simulink model "part_m"  (R2022b)
settings: Solver=ode4  StartTime=0.0  StopTime=inf  FixedStep=0.002  RelTol=1e-3
InitFcn:
  | init; % init script
values from neighbouring files (symbols this model uses):
  attitude_m0 = [theta_m0; psi_m0]    [init.m]
  attitude_t0 = [theta_t0; psi_t0]    [init.m]
  d_state_m = T_VG_m'*[V_m0;0;0;]    [init.m]
  d_state_t = T_VG_t'*[V_t0;0;0;]    [init.m]
  k_epsilon_lead_angle = k(1)    [init.m]
  k_sigma_lead_angle = k(2)    [init.m]
  state_m0 = [x_m0; y_m0; z_m0]    [init.m]
  state_t0 = [x_t0; y_t0; z_t0]    [init.m]
libraries: simulink x3
(part 1 of 2)
settings Model: Creator=Ali  LastModifiedBy=Ali

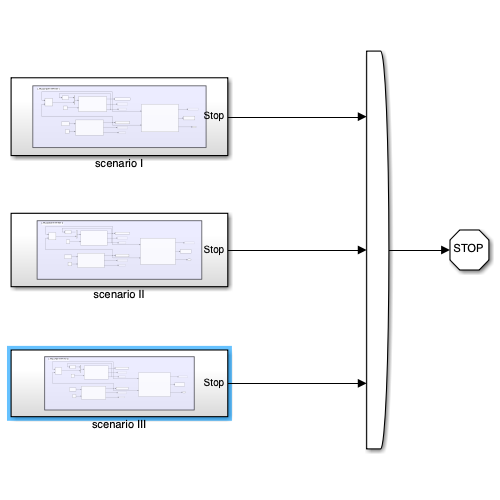
[thumbnail: Simulink's stored preview of the top-level diagram]
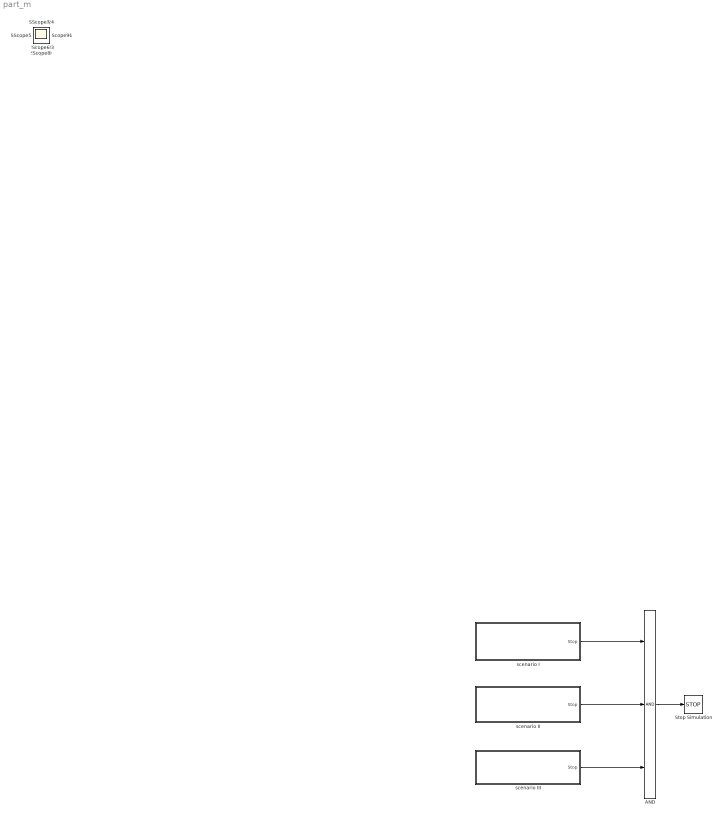
== system part_m ==
  AND : Logic  Inputs=3  IconShape=distinctive  AllPortsSameDT=off  OutDataTypeStr=boolean
  Stop Simulation : Stop
  scenario I : Subsystem
  scenario II : Subsystem
  scenario III : Subsystem
  Scope{,1..18,20..24} (24 alike) : Scope
  wires:
  scenario I/1(Stop) -> AND/1
  scenario II/1(Stop) -> AND/2
  scenario III/1(Stop) -> AND/3
  AND/1 -> Stop Simulation/1

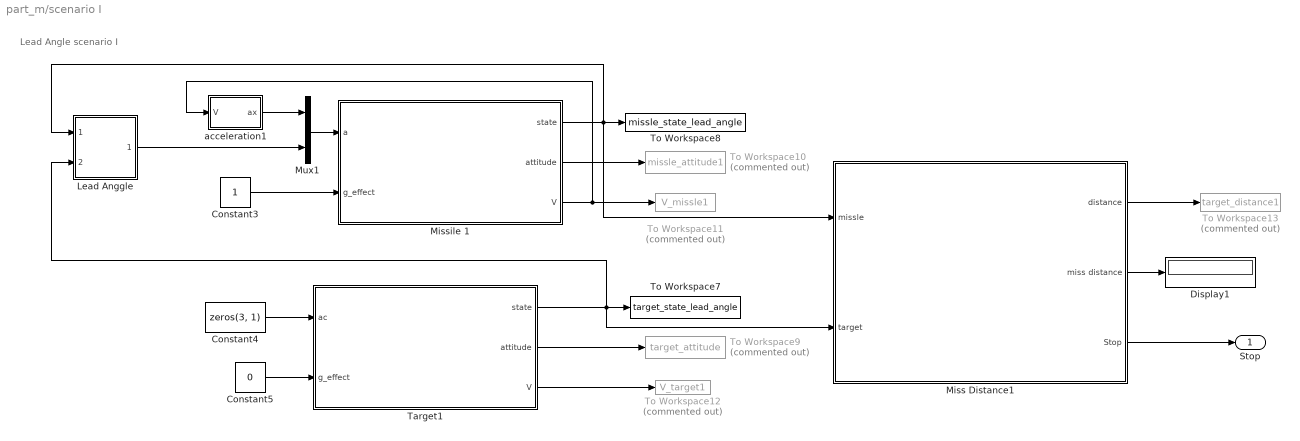
== system part_m/scenario I ==
  note: Lead Angle scenario I
  Constant3 : Constant
  Constant4 : Constant  Value=zeros(3, 1)
  Constant5 : Constant  Value=0
  Display1 : Display
  Lead Anggle : Subsystem
  Miss Distance1 : Subsystem
  Missile 1 : Subsystem
  Mux1 : Mux  Inputs=2
  Target1 : Subsystem
  To Workspace10 : ToWorkspace  Commented=on  VariableName=missle_attitude1  SaveFormat=Timeseries  SampleTime=-1
      settings: Save2DSignal=2-D array (concatenate along first dimension)
  To Workspace11 : ToWorkspace  Commented=on  VariableName=V_missle1  SaveFormat=Timeseries  SampleTime=-1
      settings: Save2DSignal=2-D array (concatenate along first dimension)
  To Workspace12 : ToWorkspace  Commented=on  VariableName=V_target1  SaveFormat=Timeseries  SampleTime=-1
      settings: Save2DSignal=2-D array (concatenate along first dimension)
  To Workspace13 : ToWorkspace  Commented=on  VariableName=target_distance1  SaveFormat=Timeseries  SampleTime=-1
      settings: Save2DSignal=2-D array (concatenate along first dimension)
  To Workspace7 : ToWorkspace  VariableName=target_state_lead_angle  SaveFormat=Timeseries  SampleTime=-1
      settings: Save2DSignal=2-D array (concatenate along first dimension)
  To Workspace8 : ToWorkspace  VariableName=missle_state_lead_angle  SaveFormat=Timeseries  SampleTime=-1
      settings: Save2DSignal=2-D array (concatenate along first dimension)
  To Workspace9 : ToWorkspace  Commented=on  VariableName=target_attitude  SaveFormat=Timeseries  SampleTime=-1
      settings: Save2DSignal=2-D array (concatenate along first dimension)
  acceleration1 : Subsystem
  Stop : Outport
  wires:
  acceleration1/1(ax) -> Mux1/1
  Miss Distance1/2(miss distance) -> Display1/1
  Constant4/1 -> Target1/1(ac)
  Constant3/1 -> Missile 1/2(g_effect)
  Lead Anggle/1("ay, az") -> Mux1/2
  Mux1/1 -> Missile 1/1(a)
  Constant5/1 -> Target1/2(g_effect)
  Missile 1/2(attitude) -> To Workspace10/1
  Target1/1(state) -> Lead Anggle/2(target_state), Miss Distance1/2(target), To Workspace7/1
  Target1/2(attitude) -> To Workspace9/1
  Missile 1/1(state) -> Lead Anggle/1(missle_state), Miss Distance1/1(missle), To Workspace8/1
  Miss Distance1/3(Stop) -> Stop/1
  Target1/3(V) -> To Workspace12/1
  Miss Distance1/1(distance) -> To Workspace13/1
  Missile 1/3(V) -> acceleration1/1(V), To Workspace11/1

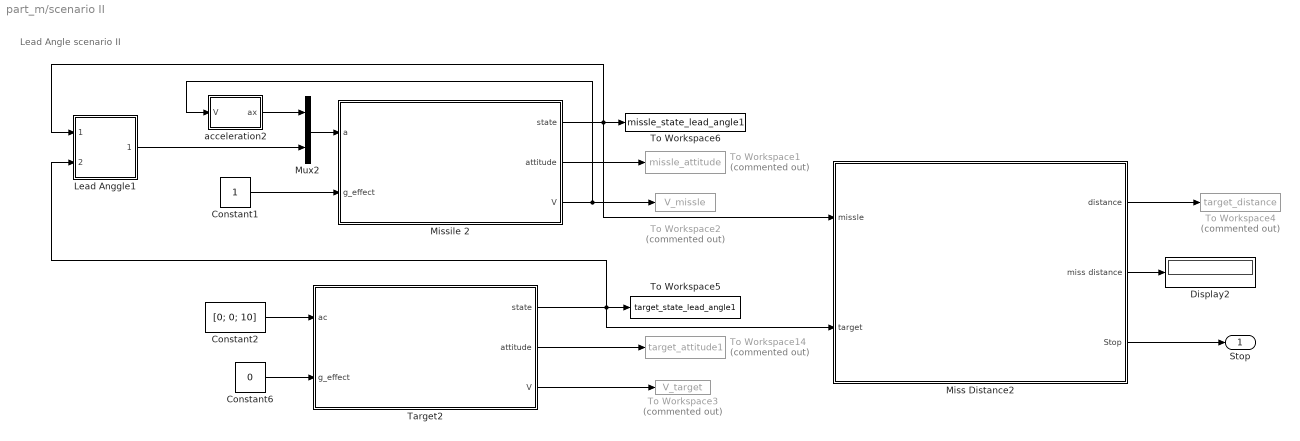
== system part_m/scenario II ==
  note: Lead Angle scenario II
  Constant1 : Constant
  Constant2 : Constant  Value=[0; 0; 10]
  Constant6 : Constant  Value=0
  Display2 : Display
  Lead Anggle1 : Subsystem
  Miss Distance2 : Subsystem
  Missile 2 : Subsystem
  Mux2 : Mux  Inputs=2
  Target2 : Subsystem
  To Workspace1 : ToWorkspace  Commented=on  VariableName=missle_attitude  SaveFormat=Timeseries  SampleTime=-1
      settings: Save2DSignal=2-D array (concatenate along first dimension)
  To Workspace14 : ToWorkspace  Commented=on  VariableName=target_attitude1  SaveFormat=Timeseries  SampleTime=-1
      settings: Save2DSignal=2-D array (concatenate along first dimension)
  To Workspace2 : ToWorkspace  Commented=on  VariableName=V_missle  SaveFormat=Timeseries  SampleTime=-1
      settings: Save2DSignal=2-D array (concatenate along first dimension)
  To Workspace3 : ToWorkspace  Commented=on  VariableName=V_target  SaveFormat=Timeseries  SampleTime=-1
      settings: Save2DSignal=2-D array (concatenate along first dimension)
  To Workspace4 : ToWorkspace  Commented=on  VariableName=target_distance  SaveFormat=Timeseries  SampleTime=-1
      settings: Save2DSignal=2-D array (concatenate along first dimension)
  To Workspace5 : ToWorkspace  VariableName=target_state_lead_angle1  SaveFormat=Timeseries  SampleTime=-1
      settings: Save2DSignal=2-D array (concatenate along first dimension)
  To Workspace6 : ToWorkspace  VariableName=missle_state_lead_angle1  SaveFormat=Timeseries  SampleTime=-1
      settings: Save2DSignal=2-D array (concatenate along first dimension)
  acceleration2 : Subsystem
  Stop : Outport
  wires:
  Constant6/1 -> Target2/2(g_effect)
  Miss Distance2/3(Stop) -> Stop/1
  Mux2/1 -> Missile 2/1(a)
  Missile 2/2(attitude) -> To Workspace1/1
  Lead Anggle1/1("ay, az") -> Mux2/2
  Constant2/1 -> Target2/1(ac)
  acceleration2/1(ax) -> Mux2/1
  Missile 2/3(V) -> acceleration2/1(V), To Workspace2/1
  Target2/2(attitude) -> To Workspace14/1
  Target2/3(V) -> To Workspace3/1
  Miss Distance2/2(miss distance) -> Display2/1
  Constant1/1 -> Missile 2/2(g_effect)
  Missile 2/1(state) -> Lead Anggle1/1(missle_state), Miss Distance2/1(missle), To Workspace6/1
  Miss Distance2/1(distance) -> To Workspace4/1
  Target2/1(state) -> Lead Anggle1/2(target_state), Miss Distance2/2(target), To Workspace5/1

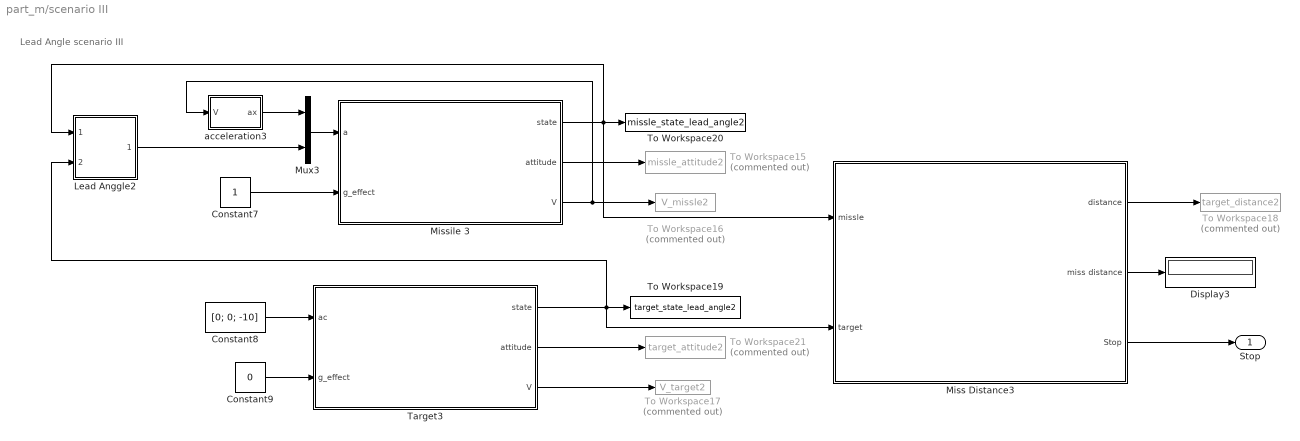
== system part_m/scenario III ==
  note: Lead Angle scenario III
  Constant7 : Constant
  Constant8 : Constant  Value=[0; 0; -10]
  Constant9 : Constant  Value=0
  Display3 : Display
  Lead Anggle2 : Subsystem
  Miss Distance3 : Subsystem
  Missile 3 : Subsystem
  Mux3 : Mux  Inputs=2
  Target3 : Subsystem
  To Workspace15 : ToWorkspace  Commented=on  VariableName=missle_attitude2  SaveFormat=Timeseries  SampleTime=-1
      settings: Save2DSignal=2-D array (concatenate along first dimension)
  To Workspace16 : ToWorkspace  Commented=on  VariableName=V_missle2  SaveFormat=Timeseries  SampleTime=-1
      settings: Save2DSignal=2-D array (concatenate along first dimension)
  To Workspace17 : ToWorkspace  Commented=on  VariableName=V_target2  SaveFormat=Timeseries  SampleTime=-1
      settings: Save2DSignal=2-D array (concatenate along first dimension)
  To Workspace18 : ToWorkspace  Commented=on  VariableName=target_distance2  SaveFormat=Timeseries  SampleTime=-1
      settings: Save2DSignal=2-D array (concatenate along first dimension)
  To Workspace19 : ToWorkspace  VariableName=target_state_lead_angle2  SaveFormat=Timeseries  SampleTime=-1
      settings: Save2DSignal=2-D array (concatenate along first dimension)
  To Workspace20 : ToWorkspace  VariableName=missle_state_lead_angle2  SaveFormat=Timeseries  SampleTime=-1
      settings: Save2DSignal=2-D array (concatenate along first dimension)
  To Workspace21 : ToWorkspace  Commented=on  VariableName=target_attitude2  SaveFormat=Timeseries  SampleTime=-1
      settings: Save2DSignal=2-D array (concatenate along first dimension)
  acceleration3 : Subsystem
  Stop : Outport
  wires:
  Miss Distance3/3(Stop) -> Stop/1
  Miss Distance3/1(distance) -> To Workspace18/1
  Target3/3(V) -> To Workspace17/1
  Target3/1(state) -> Lead Anggle2/2(target_state), Miss Distance3/2(target), To Workspace19/1
  acceleration3/1(ax) -> Mux3/1
  Target3/2(attitude) -> To Workspace21/1
  Missile 3/2(attitude) -> To Workspace15/1
  Lead Anggle2/1("ay, az") -> Mux3/2
  Missile 3/1(state) -> Lead Anggle2/1(missle_state), Miss Distance3/1(missle), To Workspace20/1
  Constant7/1 -> Missile 3/2(g_effect)
  Constant9/1 -> Target3/2(g_effect)
  Missile 3/3(V) -> acceleration3/1(V), To Workspace16/1
  Miss Distance3/2(miss distance) -> Display3/1
  Constant8/1 -> Target3/1(ac)
  Mux3/1 -> Missile 3/1(a)

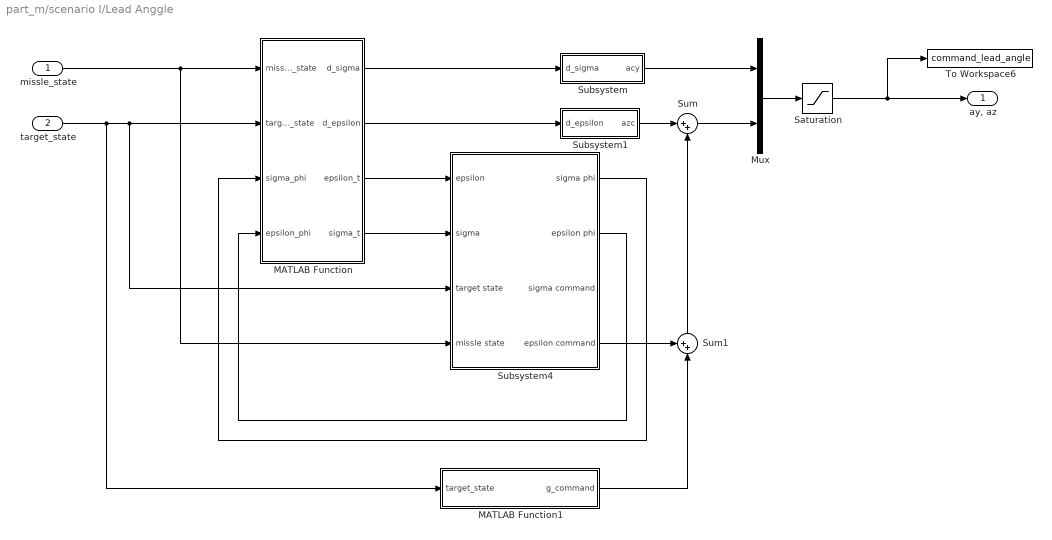
== system part_m/scenario I/Lead Anggle ==
  missle_state : Inport
  target_state : Inport  Port=2
  MATLAB Function : MATLAB Function  TreatAsAtomicUnit=on
  MATLAB Function1 : MATLAB Function  TreatAsAtomicUnit=on
  Mux : Mux  Inputs=2
  Saturation : Saturate  UpperLimit=5*9.81  LowerLimit=-5*9.81
  Subsystem : Subsystem
  Subsystem1 : Subsystem
  Subsystem4 : Subsystem
  Sum : Sum  Inputs=|++
  Sum1 : Sum  Inputs=++|
  To Workspace6 : ToWorkspace  VariableName=command_lead_angle  SaveFormat=Timeseries  SampleTime=-1
      settings: Save2DSignal=2-D array (concatenate along first dimension)
  "ay, az" : Outport
  wires:
  missle_state/1 -> Subsystem4/4(missle state), MATLAB Function/1(missle_state)
  target_state/1 -> MATLAB Function1/1(target_state), Subsystem4/3(target state), MATLAB Function/2(target_state)
  MATLAB Function/1(d_sigma) -> Subsystem/1(d_sigma)
  MATLAB Function/2(d_epsilon) -> Subsystem1/1(d_epsilon)
  Subsystem1/1(azc) -> Sum/1
  Mux/1 -> Saturation/1
  Saturation/1 -> "ay, az"/1, To Workspace6/1
  Subsystem/1(acy) -> Mux/1
  Sum/1 -> Mux/2
  MATLAB Function/3(epsilon_t) -> Subsystem4/1(epsilon)
  MATLAB Function/4(sigma_t) -> Subsystem4/2(sigma)
  Subsystem4/1(sigma phi) -> MATLAB Function/3(sigma_phi)
  Subsystem4/2(epsilon phi) -> MATLAB Function/4(epsilon_phi)
  Sum1/1 -> Sum/2
  MATLAB Function1/1(g_command) -> Sum1/2
  Subsystem4/4(epsilon command) -> Sum1/1

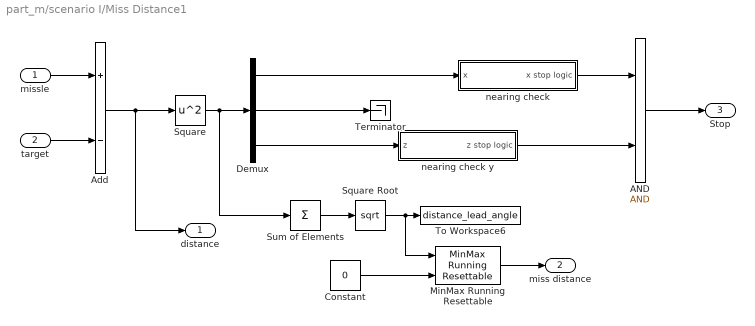
== system part_m/scenario I/Miss Distance1 ==
  missle : Inport
  target : Inport  Port=2
  AND : Logic  IconShape=distinctive  AllPortsSameDT=off  OutDataTypeStr=boolean
  Add : Sum  Inputs=+-
  Constant : Constant  Value=0
  Demux : Demux  Outputs=3
  MinMax Running Resettable : simulink/Math Operations/MinMax Running Resettable  Function=min  vinit=inf
  Square : Math  Operator=square
  Square Root : Sqrt
  Sum of Elements : Sum  Inputs=+
  Terminator : Terminator
  To Workspace6 : ToWorkspace  VariableName=distance_lead_angle  SaveFormat=Timeseries  SampleTime=-1
      settings: Save2DSignal=2-D array (concatenate along first dimension)
  nearing check : Subsystem
  nearing check y : Subsystem
  distance : Outport
  miss distance : Outport  Port=2
  Stop : Outport  Port=3
  wires:
  missle/1 -> Add/1
  Add/1 -> distance/1, Square/1
  target/1 -> Add/2
  Square/1 -> Sum of Elements/1, Demux/1
  nearing check/1(x stop logic) -> AND/1
  AND/1 -> Stop/1
  Demux/2 -> Terminator/1
  nearing check y/1(z stop logic) -> AND/2
  Sum of Elements/1 -> Square Root/1
  Square Root/1 -> MinMax Running Resettable/1, To Workspace6/1
  Demux/3 -> nearing check y/1(z)
  Demux/1 -> nearing check/1(x)
  Constant/1 -> MinMax Running Resettable/2
  MinMax Running Resettable/1 -> miss distance/1

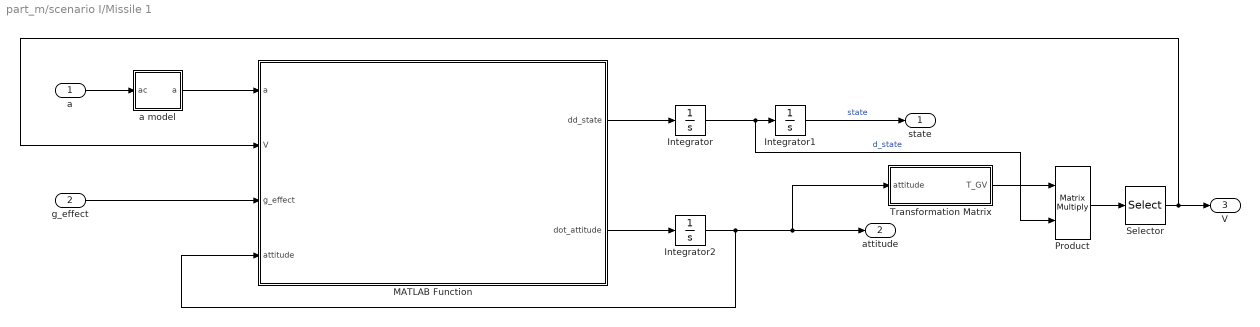
== system part_m/scenario I/Missile 1 ==
  a : Inport
  g_effect : Inport  Port=2
  Integrator : Integrator  InitialCondition=d_state_m
  Integrator1 : Integrator  InitialCondition=state_m0
  Integrator2 : Integrator  InitialCondition=attitude_m0
  MATLAB Function : MATLAB Function  TreatAsAtomicUnit=on
  Product : Product  Multiplication=Matrix(*)
  Selector : Selector  InputPortWidth=3  IndexOptions=Index vector (dialog)  Indices=[1]  OutputSizes=1
  Transformation Matrix : MATLAB Function  TreatAsAtomicUnit=on
  a model : Subsystem
  state : Outport
  attitude : Outport  Port=2
  V : Outport  Port=3
  wires:
  MATLAB Function/2(dot_attitude) -> Integrator2/1
  Integrator1/1 -> state/1  "state"
  MATLAB Function/1(dd_state) -> Integrator/1
  g_effect/1 -> MATLAB Function/3(g_effect)
  Integrator/1 -> Product/2, Integrator1/1  "d_state"
  Product/1 -> Selector/1
  Selector/1 -> MATLAB Function/2(V), V/1
  Transformation Matrix/1(T_GV) -> Product/1
  Integrator2/1 -> Transformation Matrix/1(attitude), attitude/1, MATLAB Function/4(attitude)
  a/1 -> a model/1(ac)
  a model/1(a) -> MATLAB Function/1(a)

== system part_m/scenario I/Target1 ==
  ac : Inport
  g_effect : Inport  Port=2
  Integrator : Integrator  InitialCondition=d_state_t
  Integrator1 : Integrator  InitialCondition=state_t0
  Integrator2 : Integrator  InitialCondition=attitude_t0
  MATLAB Function : MATLAB Function  TreatAsAtomicUnit=on
  Product : Product  Multiplication=Matrix(*)
  Selector : Selector  InputPortWidth=3  IndexOptions=Index vector (dialog)  Indices=[1]  OutputSizes=1
  Transformation Matrix : MATLAB Function  TreatAsAtomicUnit=on
  state : Outport
  attitude : Outport  Port=2
  V : Outport  Port=3
  wires:
  MATLAB Function/2(dot_attitude) -> Integrator2/1
  Integrator1/1 -> state/1  "state"
  MATLAB Function/1(dd_state) -> Integrator/1
  g_effect/1 -> MATLAB Function/3(g_effect)
  Integrator/1 -> Product/2, Integrator1/1  "d_state"
  Integrator2/1 -> MATLAB Function/4(attitude), Transformation Matrix/1(attitude), attitude/1
  Product/1 -> Selector/1
  Selector/1 -> MATLAB Function/2(V), V/1
  Transformation Matrix/1(T_GV) -> Product/1
  ac/1 -> MATLAB Function/1(a)

== system part_m/scenario I/acceleration1 ==
  V : Inport
  Add : Sum
  Add1 : Sum  Inputs=+-
  Constant1 : Constant  Value=1.5e-4
  Gain : Gain  Gain=300
  Product : Product
  Square : Math  Operator=square
  Step : Step  Time=3  After=-1  SampleTime=0
  Step1 : Step  Time=0  SampleTime=0
  ax : Outport
  wires:
  V/1 -> Square/1
  Step/1 -> Add/1
  Square/1 -> Product/2
  Constant1/1 -> Product/1
  Add1/1 -> ax/1
  Step1/1 -> Add/2
  Gain/1 -> Add1/1
  Add/1 -> Gain/1
  Product/1 -> Add1/2

== system part_m/scenario II/Lead Anggle1 ==
  missle_state : Inport
  target_state : Inport  Port=2
  MATLAB Function : MATLAB Function  TreatAsAtomicUnit=on
  MATLAB Function1 : MATLAB Function  TreatAsAtomicUnit=on
  Mux : Mux  Inputs=2
  Saturation : Saturate  UpperLimit=5*9.81  LowerLimit=-5*9.81
  Subsystem : Subsystem
  Subsystem1 : Subsystem
  Subsystem4 : Subsystem
  Sum : Sum  Inputs=|++
  Sum1 : Sum  Inputs=++|
  To Workspace6 : ToWorkspace  VariableName=command_lead_angle1  SaveFormat=Timeseries  SampleTime=-1
      settings: Save2DSignal=2-D array (concatenate along first dimension)
  "ay, az" : Outport
  wires:
  missle_state/1 -> Subsystem4/4(missle state), MATLAB Function/1(missle_state)
  target_state/1 -> MATLAB Function1/1(target_state), Subsystem4/3(target state), MATLAB Function/2(target_state)
  MATLAB Function/1(d_sigma) -> Subsystem/1(d_sigma)
  MATLAB Function/2(d_epsilon) -> Subsystem1/1(d_epsilon)
  Subsystem1/1(azc) -> Sum/1
  Mux/1 -> Saturation/1
  Saturation/1 -> "ay, az"/1, To Workspace6/1
  Subsystem/1(acy) -> Mux/1
  Sum/1 -> Mux/2
  MATLAB Function/3(epsilon_t) -> Subsystem4/1(epsilon)
  MATLAB Function/4(sigma_t) -> Subsystem4/2(sigma)
  Subsystem4/1(sigma phi) -> MATLAB Function/3(sigma_phi)
  Subsystem4/2(epsilon phi) -> MATLAB Function/4(epsilon_phi)
  Sum1/1 -> Sum/2
  MATLAB Function1/1(g_command) -> Sum1/2
  Subsystem4/4(epsilon command) -> Sum1/1

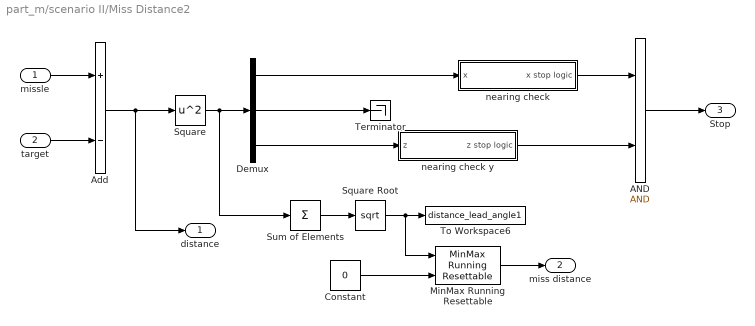
== system part_m/scenario II/Miss Distance2 ==
  missle : Inport
  target : Inport  Port=2
  AND : Logic  IconShape=distinctive  AllPortsSameDT=off  OutDataTypeStr=boolean
  Add : Sum  Inputs=+-
  Constant : Constant  Value=0
  Demux : Demux  Outputs=3
  MinMax Running Resettable : simulink/Math Operations/MinMax Running Resettable  Function=min  vinit=inf
  Square : Math  Operator=square
  Square Root : Sqrt
  Sum of Elements : Sum  Inputs=+
  Terminator : Terminator
  To Workspace6 : ToWorkspace  VariableName=distance_lead_angle1  SaveFormat=Timeseries  SampleTime=-1
      settings: Save2DSignal=2-D array (concatenate along first dimension)
  nearing check : Subsystem
  nearing check y : Subsystem
  distance : Outport
  miss distance : Outport  Port=2
  Stop : Outport  Port=3
  wires:
  missle/1 -> Add/1
  Add/1 -> distance/1, Square/1
  target/1 -> Add/2
  Square/1 -> Sum of Elements/1, Demux/1
  nearing check/1(x stop logic) -> AND/1
  AND/1 -> Stop/1
  Demux/2 -> Terminator/1
  nearing check y/1(z stop logic) -> AND/2
  Sum of Elements/1 -> Square Root/1
  Square Root/1 -> MinMax Running Resettable/1, To Workspace6/1
  Demux/3 -> nearing check y/1(z)
  Demux/1 -> nearing check/1(x)
  Constant/1 -> MinMax Running Resettable/2
  MinMax Running Resettable/1 -> miss distance/1

== system part_m/scenario II/Missile 2 ==
  a : Inport
  g_effect : Inport  Port=2
  Integrator : Integrator  InitialCondition=d_state_m
  Integrator1 : Integrator  InitialCondition=state_m0
  Integrator2 : Integrator  InitialCondition=attitude_m0
  MATLAB Function : MATLAB Function  TreatAsAtomicUnit=on
  Product : Product  Multiplication=Matrix(*)
  Selector : Selector  InputPortWidth=3  IndexOptions=Index vector (dialog)  Indices=[1]  OutputSizes=1
  Transformation Matrix : MATLAB Function  TreatAsAtomicUnit=on
  a model : Subsystem
  state : Outport
  attitude : Outport  Port=2
  V : Outport  Port=3
  wires:
  MATLAB Function/2(dot_attitude) -> Integrator2/1
  Integrator1/1 -> state/1  "state"
  MATLAB Function/1(dd_state) -> Integrator/1
  g_effect/1 -> MATLAB Function/3(g_effect)
  Integrator/1 -> Product/2, Integrator1/1  "d_state"
  Product/1 -> Selector/1
  Selector/1 -> MATLAB Function/2(V), V/1
  Transformation Matrix/1(T_GV) -> Product/1
  Integrator2/1 -> Transformation Matrix/1(attitude), attitude/1, MATLAB Function/4(attitude)
  a/1 -> a model/1(ac)
  a model/1(a) -> MATLAB Function/1(a)

== system part_m/scenario II/Target2 ==
  ac : Inport
  g_effect : Inport  Port=2
  Integrator : Integrator  InitialCondition=d_state_t
  Integrator1 : Integrator  InitialCondition=state_t0
  Integrator2 : Integrator  InitialCondition=attitude_t0
  MATLAB Function : MATLAB Function  TreatAsAtomicUnit=on
  Product : Product  Multiplication=Matrix(*)
  Selector : Selector  InputPortWidth=3  IndexOptions=Index vector (dialog)  Indices=[1]  OutputSizes=1
  Transformation Matrix : MATLAB Function  TreatAsAtomicUnit=on
  state : Outport
  attitude : Outport  Port=2
  V : Outport  Port=3
  wires:
  MATLAB Function/2(dot_attitude) -> Integrator2/1
  Integrator1/1 -> state/1  "state"
  MATLAB Function/1(dd_state) -> Integrator/1
  g_effect/1 -> MATLAB Function/3(g_effect)
  Integrator/1 -> Product/2, Integrator1/1  "d_state"
  Integrator2/1 -> MATLAB Function/4(attitude), Transformation Matrix/1(attitude), attitude/1
  Product/1 -> Selector/1
  Selector/1 -> MATLAB Function/2(V), V/1
  Transformation Matrix/1(T_GV) -> Product/1
  ac/1 -> MATLAB Function/1(a)

== system part_m/scenario II/acceleration2 ==
  V : Inport
  Add : Sum
  Add1 : Sum  Inputs=+-
  Constant1 : Constant  Value=1.5e-4
  Gain : Gain  Gain=300
  Product : Product
  Square : Math  Operator=square
  Step : Step  Time=3  After=-1  SampleTime=0
  Step1 : Step  Time=0  SampleTime=0
  ax : Outport
  wires:
  V/1 -> Square/1
  Step/1 -> Add/1
  Square/1 -> Product/2
  Constant1/1 -> Product/1
  Add1/1 -> ax/1
  Step1/1 -> Add/2
  Gain/1 -> Add1/1
  Add/1 -> Gain/1
  Product/1 -> Add1/2

== system part_m/scenario III/Lead Anggle2 ==
  missle_state : Inport
  target_state : Inport  Port=2
  MATLAB Function : MATLAB Function  TreatAsAtomicUnit=on
  MATLAB Function1 : MATLAB Function  TreatAsAtomicUnit=on
  Mux : Mux  Inputs=2
  Saturation : Saturate  UpperLimit=5*9.81  LowerLimit=-5*9.81
  Subsystem : Subsystem
  Subsystem1 : Subsystem
  Subsystem4 : Subsystem
  Sum : Sum  Inputs=|++
  Sum1 : Sum  Inputs=++|
  To Workspace6 : ToWorkspace  VariableName=command_lead_angle2  SaveFormat=Timeseries  SampleTime=-1
      settings: Save2DSignal=2-D array (concatenate along first dimension)
  "ay, az" : Outport
  wires:
  missle_state/1 -> Subsystem4/4(missle state), MATLAB Function/1(missle_state)
  target_state/1 -> MATLAB Function1/1(target_state), Subsystem4/3(target state), MATLAB Function/2(target_state)
  MATLAB Function/1(d_sigma) -> Subsystem/1(d_sigma)
  MATLAB Function/2(d_epsilon) -> Subsystem1/1(d_epsilon)
  Subsystem1/1(azc) -> Sum/1
  Mux/1 -> Saturation/1
  Saturation/1 -> "ay, az"/1, To Workspace6/1
  Subsystem/1(acy) -> Mux/1
  Sum/1 -> Mux/2
  MATLAB Function/3(epsilon_t) -> Subsystem4/1(epsilon)
  MATLAB Function/4(sigma_t) -> Subsystem4/2(sigma)
  Subsystem4/1(sigma phi) -> MATLAB Function/3(sigma_phi)
  Subsystem4/2(epsilon phi) -> MATLAB Function/4(epsilon_phi)
  Sum1/1 -> Sum/2
  MATLAB Function1/1(g_command) -> Sum1/2
  Subsystem4/4(epsilon command) -> Sum1/1

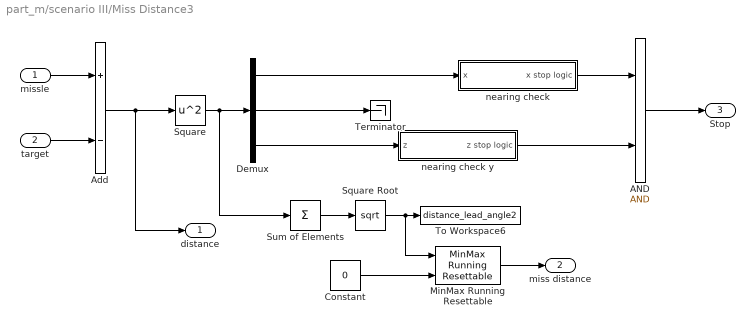
== system part_m/scenario III/Miss Distance3 ==
  missle : Inport
  target : Inport  Port=2
  AND : Logic  IconShape=distinctive  AllPortsSameDT=off  OutDataTypeStr=boolean
  Add : Sum  Inputs=+-
  Constant : Constant  Value=0
  Demux : Demux  Outputs=3
  MinMax Running Resettable : simulink/Math Operations/MinMax Running Resettable  Function=min  vinit=inf
  Square : Math  Operator=square
  Square Root : Sqrt
  Sum of Elements : Sum  Inputs=+
  Terminator : Terminator
  To Workspace6 : ToWorkspace  VariableName=distance_lead_angle2  SaveFormat=Timeseries  SampleTime=-1
      settings: Save2DSignal=2-D array (concatenate along first dimension)
  nearing check : Subsystem
  nearing check y : Subsystem
  distance : Outport
  miss distance : Outport  Port=2
  Stop : Outport  Port=3
  wires:
  missle/1 -> Add/1
  Add/1 -> distance/1, Square/1
  target/1 -> Add/2
  Square/1 -> Sum of Elements/1, Demux/1
  nearing check/1(x stop logic) -> AND/1
  AND/1 -> Stop/1
  Demux/2 -> Terminator/1
  nearing check y/1(z stop logic) -> AND/2
  Sum of Elements/1 -> Square Root/1
  Square Root/1 -> MinMax Running Resettable/1, To Workspace6/1
  Demux/3 -> nearing check y/1(z)
  Demux/1 -> nearing check/1(x)
  Constant/1 -> MinMax Running Resettable/2
  MinMax Running Resettable/1 -> miss distance/1

== system part_m/scenario III/Missile 3 ==
  a : Inport
  g_effect : Inport  Port=2
  Integrator : Integrator  InitialCondition=d_state_m
  Integrator1 : Integrator  InitialCondition=state_m0
  Integrator2 : Integrator  InitialCondition=attitude_m0
  MATLAB Function : MATLAB Function  TreatAsAtomicUnit=on
  Product : Product  Multiplication=Matrix(*)
  Selector : Selector  InputPortWidth=3  IndexOptions=Index vector (dialog)  Indices=[1]  OutputSizes=1
  Transformation Matrix : MATLAB Function  TreatAsAtomicUnit=on
  a model : Subsystem
  state : Outport
  attitude : Outport  Port=2
  V : Outport  Port=3
  wires:
  MATLAB Function/2(dot_attitude) -> Integrator2/1
  Integrator1/1 -> state/1  "state"
  MATLAB Function/1(dd_state) -> Integrator/1
  g_effect/1 -> MATLAB Function/3(g_effect)
  Integrator/1 -> Product/2, Integrator1/1  "d_state"
  Product/1 -> Selector/1
  Selector/1 -> MATLAB Function/2(V), V/1
  Transformation Matrix/1(T_GV) -> Product/1
  Integrator2/1 -> Transformation Matrix/1(attitude), attitude/1, MATLAB Function/4(attitude)
  a/1 -> a model/1(ac)
  a model/1(a) -> MATLAB Function/1(a)

== system part_m/scenario III/Target3 ==
  ac : Inport
  g_effect : Inport  Port=2
  Integrator : Integrator  InitialCondition=d_state_t
  Integrator1 : Integrator  InitialCondition=state_t0
  Integrator2 : Integrator  InitialCondition=attitude_t0
  MATLAB Function : MATLAB Function  TreatAsAtomicUnit=on
  Product : Product  Multiplication=Matrix(*)
  Selector : Selector  InputPortWidth=3  IndexOptions=Index vector (dialog)  Indices=[1]  OutputSizes=1
  Transformation Matrix : MATLAB Function  TreatAsAtomicUnit=on
  state : Outport
  attitude : Outport  Port=2
  V : Outport  Port=3
  wires:
  MATLAB Function/2(dot_attitude) -> Integrator2/1
  Integrator1/1 -> state/1  "state"
  MATLAB Function/1(dd_state) -> Integrator/1
  g_effect/1 -> MATLAB Function/3(g_effect)
  Integrator/1 -> Product/2, Integrator1/1  "d_state"
  Integrator2/1 -> MATLAB Function/4(attitude), Transformation Matrix/1(attitude), attitude/1
  Product/1 -> Selector/1
  Selector/1 -> MATLAB Function/2(V), V/1
  Transformation Matrix/1(T_GV) -> Product/1
  ac/1 -> MATLAB Function/1(a)

== system part_m/scenario III/acceleration3 ==
  V : Inport
  Add : Sum
  Add1 : Sum  Inputs=+-
  Constant1 : Constant  Value=1.5e-4
  Gain : Gain  Gain=300
  Product : Product
  Square : Math  Operator=square
  Step : Step  Time=3  After=-1  SampleTime=0
  Step1 : Step  Time=0  SampleTime=0
  ax : Outport
  wires:
  V/1 -> Square/1
  Step/1 -> Add/1
  Square/1 -> Product/2
  Constant1/1 -> Product/1
  Add1/1 -> ax/1
  Step1/1 -> Add/2
  Gain/1 -> Add1/1
  Add/1 -> Gain/1
  Product/1 -> Add1/2

== system part_m/scenario I/Lead Anggle/Subsystem ==
  d_sigma : Inport
  Gain : Gain  Gain=k_sigma_lead_angle
  Sum : Sum  Inputs=+|+
  Transfer Fcn : TransferFcn  Numerator=[1000 0]  Denominator=[1 100]
  acy : Outport
  wires:
  d_sigma/1 -> Gain/1, Transfer Fcn/1
  Transfer Fcn/1 -> Sum/2
  Sum/1 -> acy/1
  Gain/1 -> Sum/1

== system part_m/scenario I/Lead Anggle/Subsystem1 ==
  d_epsilon : Inport
  Gain1 : Gain  Gain=k_epsilon_lead_angle
  Sum : Sum  Inputs=+|+
  Transfer Fcn : TransferFcn  Numerator=[1000 0]  Denominator=[1 100]
  azc : Outport
  wires:
  d_epsilon/1 -> Transfer Fcn/1, Gain1/1
  Gain1/1 -> Sum/1
  Transfer Fcn/1 -> Sum/2
  Sum/1 -> azc/1

== system part_m/scenario I/Lead Anggle/Subsystem4 ==
  epsilon : Inport
  sigma : Inport  Port=2
  target state : Inport  Port=3
  missle state : Inport  Port=4
  Add : Sum  Inputs=-+
  Delay : Delay  DelayLength=1
  Delay1 : Delay  DelayLength=1
  Subsystem2 : Subsystem
  Subsystem3 : Subsystem
  sigma phi : Outport
  epsilon phi : Outport  Port=2
  sigma command : Outport  Port=3
  epsilon command : Outport  Port=4
  wires:
  sigma/1 -> Subsystem3/2(sigma), Delay1/1
  epsilon/1 -> Subsystem3/1(epsilon), Delay/1
  Delay1/1 -> Subsystem2/2(sigma)
  Delay/1 -> Subsystem2/1(epsilon)
  Subsystem2/2(epsilon phi) -> epsilon phi/1
  Subsystem2/1(sigma phi) -> sigma phi/1
  target state/1 -> Add/1, Subsystem3/3(target_state)
  missle state/1 -> Add/2
  Add/1 -> Subsystem2/3(delta_state)
  Subsystem3/1(sigma command) -> sigma command/1
  Subsystem3/2(epsilon command) -> epsilon command/1

== system part_m/scenario I/Miss Distance1/nearing check ==
  x : Inport
  Add1 : Sum  Inputs=-+
  Constant3 : Constant  Value=0
  Constant4 : Constant
  Delay : Delay  DelayLength=1  InitialCondition=inf
  Switch : Switch  Criteria=u2 > Threshold  SaturateOnIntegerOverflow=off  InputSameDT=off
  x stop logic : Outport
  wires:
  Switch/1 -> x stop logic/1
  Constant3/1 -> Switch/1
  Constant4/1 -> Switch/3
  x/1 -> Delay/1, Add1/1
  Add1/1 -> Switch/2
  Delay/1 -> Add1/2

== system part_m/scenario I/Miss Distance1/nearing check y ==
  z : Inport
  Add1 : Sum  Inputs=-+
  Constant3 : Constant  Value=0
  Constant4 : Constant
  Delay : Delay  DelayLength=1  InitialCondition=inf
  Switch : Switch  Criteria=u2 > Threshold  SaturateOnIntegerOverflow=off  InputSameDT=off
  z stop logic : Outport
  wires:
  Delay/1 -> Add1/2
  Add1/1 -> Switch/2
  z/1 -> Add1/1, Delay/1
  Constant4/1 -> Switch/3
  Constant3/1 -> Switch/1
  Switch/1 -> z stop logic/1

== system part_m/scenario I/Missile 1/a model ==
  ac : Inport
  Demux : Demux  Outputs=3
  Mux : Mux  Inputs=3
  Transfer Fcn : TransferFcn  Numerator=[30 200]  Denominator=[1 30 200]
  Transfer Fcn1 : TransferFcn  Numerator=[30 200]  Denominator=[1 30 200]
  a : Outport
  wires:
  Transfer Fcn/1 -> Mux/2
  Mux/1 -> a/1
  Transfer Fcn1/1 -> Mux/3
  Demux/2 -> Transfer Fcn/1
  Demux/3 -> Transfer Fcn1/1
  Demux/1 -> Mux/1
  ac/1 -> Demux/1

== system part_m/scenario II/Lead Anggle1/Subsystem ==
  d_sigma : Inport
  Gain : Gain  Gain=k_sigma_lead_angle
  Sum : Sum  Inputs=+|+
  Transfer Fcn : TransferFcn  Numerator=[1000 0]  Denominator=[1 100]
  acy : Outport
  wires:
  d_sigma/1 -> Gain/1, Transfer Fcn/1
  Transfer Fcn/1 -> Sum/2
  Sum/1 -> acy/1
  Gain/1 -> Sum/1

== system part_m/scenario II/Lead Anggle1/Subsystem1 ==
  d_epsilon : Inport
  Gain1 : Gain  Gain=k_epsilon_lead_angle
  Sum : Sum  Inputs=+|+
  Transfer Fcn : TransferFcn  Numerator=[1000 0]  Denominator=[1 100]
  azc : Outport
  wires:
  d_epsilon/1 -> Transfer Fcn/1, Gain1/1
  Gain1/1 -> Sum/1
  Transfer Fcn/1 -> Sum/2
  Sum/1 -> azc/1

== system part_m/scenario II/Lead Anggle1/Subsystem4 ==
  epsilon : Inport
  sigma : Inport  Port=2
  target state : Inport  Port=3
  missle state : Inport  Port=4
  Add : Sum  Inputs=-+
  Delay : Delay  DelayLength=1
  Delay1 : Delay  DelayLength=1
  Subsystem2 : Subsystem
  Subsystem3 : Subsystem
  sigma phi : Outport
  epsilon phi : Outport  Port=2
  sigma command : Outport  Port=3
  epsilon command : Outport  Port=4
  wires:
  sigma/1 -> Subsystem3/2(sigma), Delay1/1
  epsilon/1 -> Subsystem3/1(epsilon), Delay/1
  Delay1/1 -> Subsystem2/2(sigma)
  Delay/1 -> Subsystem2/1(epsilon)
  Subsystem2/2(epsilon phi) -> epsilon phi/1
  Subsystem2/1(sigma phi) -> sigma phi/1
  target state/1 -> Add/1, Subsystem3/3(target_state)
  missle state/1 -> Add/2
  Add/1 -> Subsystem2/3(delta_state)
  Subsystem3/1(sigma command) -> sigma command/1
  Subsystem3/2(epsilon command) -> epsilon command/1

== system part_m/scenario II/Miss Distance2/nearing check ==
  x : Inport
  Add1 : Sum  Inputs=-+
  Constant3 : Constant  Value=0
  Constant4 : Constant
  Delay : Delay  DelayLength=1  InitialCondition=inf
  Switch : Switch  Criteria=u2 > Threshold  SaturateOnIntegerOverflow=off  InputSameDT=off
  x stop logic : Outport
  wires:
  Switch/1 -> x stop logic/1
  Constant3/1 -> Switch/1
  Constant4/1 -> Switch/3
  x/1 -> Delay/1, Add1/1
  Add1/1 -> Switch/2
  Delay/1 -> Add1/2

== system part_m/scenario II/Miss Distance2/nearing check y ==
  z : Inport
  Add1 : Sum  Inputs=-+
  Constant3 : Constant  Value=0
  Constant4 : Constant
  Delay : Delay  DelayLength=1  InitialCondition=inf
  Switch : Switch  Criteria=u2 > Threshold  SaturateOnIntegerOverflow=off  InputSameDT=off
  z stop logic : Outport
  wires:
  Delay/1 -> Add1/2
  Add1/1 -> Switch/2
  z/1 -> Add1/1, Delay/1
  Constant4/1 -> Switch/3
  Constant3/1 -> Switch/1
  Switch/1 -> z stop logic/1

== system part_m/scenario II/Missile 2/a model ==
  ac : Inport
  Demux : Demux  Outputs=3
  Mux : Mux  Inputs=3
  Transfer Fcn : TransferFcn  Numerator=[30 200]  Denominator=[1 30 200]
  Transfer Fcn1 : TransferFcn  Numerator=[30 200]  Denominator=[1 30 200]
  a : Outport
  wires:
  Transfer Fcn/1 -> Mux/2
  Mux/1 -> a/1
  Transfer Fcn1/1 -> Mux/3
  Demux/2 -> Transfer Fcn/1
  Demux/3 -> Transfer Fcn1/1
  Demux/1 -> Mux/1
  ac/1 -> Demux/1

== system part_m/scenario III/Lead Anggle2/Subsystem ==
  d_sigma : Inport
  Gain : Gain  Gain=k_sigma_lead_angle
  Sum : Sum  Inputs=+|+
  Transfer Fcn : TransferFcn  Numerator=[1000 0]  Denominator=[1 100]
  acy : Outport
  wires:
  d_sigma/1 -> Gain/1, Transfer Fcn/1
  Transfer Fcn/1 -> Sum/2
  Sum/1 -> acy/1
  Gain/1 -> Sum/1

== system part_m/scenario III/Lead Anggle2/Subsystem1 ==
  d_epsilon : Inport
  Gain1 : Gain  Gain=k_epsilon_lead_angle
  Sum : Sum  Inputs=+|+
  Transfer Fcn : TransferFcn  Numerator=[1000 0]  Denominator=[1 100]
  azc : Outport
  wires:
  d_epsilon/1 -> Transfer Fcn/1, Gain1/1
  Gain1/1 -> Sum/1
  Transfer Fcn/1 -> Sum/2
  Sum/1 -> azc/1

== system part_m/scenario III/Lead Anggle2/Subsystem4 ==
  epsilon : Inport
  sigma : Inport  Port=2
  target state : Inport  Port=3
  missle state : Inport  Port=4
  Add : Sum  Inputs=-+
  Delay : Delay  DelayLength=1
  Delay1 : Delay  DelayLength=1
  Subsystem2 : Subsystem
  Subsystem3 : Subsystem
  sigma phi : Outport
  epsilon phi : Outport  Port=2
  sigma command : Outport  Port=3
  epsilon command : Outport  Port=4
  wires:
  sigma/1 -> Subsystem3/2(sigma), Delay1/1
  epsilon/1 -> Subsystem3/1(epsilon), Delay/1
  Delay1/1 -> Subsystem2/2(sigma)
  Delay/1 -> Subsystem2/1(epsilon)
  Subsystem2/2(epsilon phi) -> epsilon phi/1
  Subsystem2/1(sigma phi) -> sigma phi/1
  target state/1 -> Add/1, Subsystem3/3(target_state)
  missle state/1 -> Add/2
  Add/1 -> Subsystem2/3(delta_state)
  Subsystem3/1(sigma command) -> sigma command/1
  Subsystem3/2(epsilon command) -> epsilon command/1

== system part_m/scenario III/Miss Distance3/nearing check ==
  x : Inport
  Add1 : Sum  Inputs=-+
  Constant3 : Constant  Value=0
  Constant4 : Constant
  Delay : Delay  DelayLength=1  InitialCondition=inf
  Switch : Switch  Criteria=u2 > Threshold  SaturateOnIntegerOverflow=off  InputSameDT=off
  x stop logic : Outport
  wires:
  Switch/1 -> x stop logic/1
  Constant3/1 -> Switch/1
  Constant4/1 -> Switch/3
  x/1 -> Delay/1, Add1/1
  Add1/1 -> Switch/2
  Delay/1 -> Add1/2

== system part_m/scenario III/Miss Distance3/nearing check y ==
  z : Inport
  Add1 : Sum  Inputs=-+
  Constant3 : Constant  Value=0
  Constant4 : Constant
  Delay : Delay  DelayLength=1  InitialCondition=inf
  Switch : Switch  Criteria=u2 > Threshold  SaturateOnIntegerOverflow=off  InputSameDT=off
  z stop logic : Outport
  wires:
  Delay/1 -> Add1/2
  Add1/1 -> Switch/2
  z/1 -> Add1/1, Delay/1
  Constant4/1 -> Switch/3
  Constant3/1 -> Switch/1
  Switch/1 -> z stop logic/1

== system part_m/scenario III/Missile 3/a model ==
  ac : Inport
  Demux : Demux  Outputs=3
  Mux : Mux  Inputs=3
  Transfer Fcn : TransferFcn  Numerator=[30 200]  Denominator=[1 30 200]
  Transfer Fcn1 : TransferFcn  Numerator=[30 200]  Denominator=[1 30 200]
  a : Outport
  wires:
  Transfer Fcn/1 -> Mux/2
  Mux/1 -> a/1
  Transfer Fcn1/1 -> Mux/3
  Demux/2 -> Transfer Fcn/1
  Demux/3 -> Transfer Fcn1/1
  Demux/1 -> Mux/1
  ac/1 -> Demux/1

== system part_m/scenario I/Lead Anggle/Subsystem4/Subsystem2 ==
  epsilon : Inport
  sigma : Inport  Port=2
  delta_state : Inport  Port=3
  MATLAB Function : MATLAB Function  TreatAsAtomicUnit=on
  Product : Product  Multiplication=Matrix(*)
  Sqrt : Sqrt
  Transfer Fcn : TransferFcn  Numerator=[100 0]  Denominator=[1 100]
  Transfer Fcn2 : TransferFcn  Numerator=[100 0]  Denominator=[1 100]
  Transfer Fcn4 : TransferFcn  Numerator=[100 0]  Denominator=[1 100]
  Transpose : Math  Operator=transpose
  sigma phi : Outport
  epsilon phi : Outport  Port=2
  wires:
  sigma/1 -> Transfer Fcn/1
  Transfer Fcn/1 -> MATLAB Function/1(d_sigma)  "d_sigma"
  epsilon/1 -> Transfer Fcn2/1
  Transfer Fcn2/1 -> MATLAB Function/4(d_epsilon)  "d_epsilon"
  delta_state/1 -> Product/2, Transpose/1
  Product/1 -> Sqrt/1
  Transpose/1 -> Product/1
  Sqrt/1 -> MATLAB Function/3(delta_R), Transfer Fcn4/1  "R_m"
  Transfer Fcn4/1 -> MATLAB Function/2(d_delta_R)  "d_R_m"
  MATLAB Function/1(epsilon_phi) -> epsilon phi/1
  MATLAB Function/2(sigma_phi) -> sigma phi/1

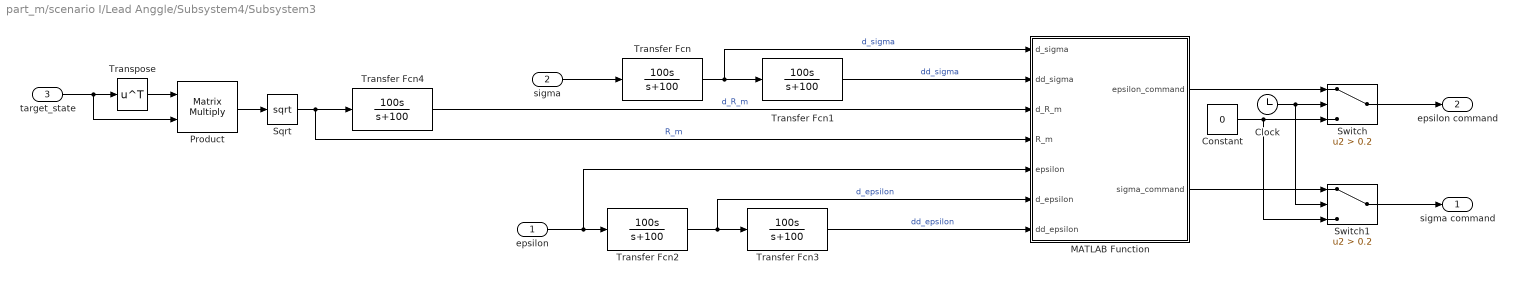
== system part_m/scenario I/Lead Anggle/Subsystem4/Subsystem3 ==
  epsilon : Inport
  sigma : Inport  Port=2
  target_state : Inport  Port=3
  Clock : Clock
  Constant : Constant  Value=0
  MATLAB Function : MATLAB Function  TreatAsAtomicUnit=on
  Product : Product  Multiplication=Matrix(*)
  Sqrt : Sqrt
  Switch : Switch  Criteria=u2 > Threshold  Threshold=0.2  SaturateOnIntegerOverflow=off  InputSameDT=off
  Switch1 : Switch  Criteria=u2 > Threshold  Threshold=0.2  SaturateOnIntegerOverflow=off  InputSameDT=off
  Transfer Fcn{,1..4} (5 alike) : TransferFcn  Numerator=[100 0]  Denominator=[1 100]
  Transpose : Math  Operator=transpose
  sigma command : Outport
  epsilon command : Outport  Port=2
  wires:
  sigma/1 -> Transfer Fcn/1
  Transfer Fcn1/1 -> MATLAB Function/2(dd_sigma)  "dd_sigma"
  Transfer Fcn/1 -> MATLAB Function/1(d_sigma), Transfer Fcn1/1  "d_sigma"
  epsilon/1 -> MATLAB Function/5(epsilon), Transfer Fcn2/1
  Transfer Fcn2/1 -> MATLAB Function/6(d_epsilon), Transfer Fcn3/1  "d_epsilon"
  target_state/1 -> Product/2, Transpose/1
  Product/1 -> Sqrt/1
  Transpose/1 -> Product/1
  Sqrt/1 -> MATLAB Function/4(R_m), Transfer Fcn4/1  "R_m"
  Transfer Fcn3/1 -> MATLAB Function/7(dd_epsilon)  "dd_epsilon"
  Transfer Fcn4/1 -> MATLAB Function/3(d_R_m)  "d_R_m"
  Clock/1 -> Switch1/2, Switch/2
  Switch/1 -> epsilon command/1
  MATLAB Function/1(epsilon_command) -> Switch/1
  Constant/1 -> Switch1/3, Switch/3
  Switch1/1 -> sigma command/1
  MATLAB Function/2(sigma_command) -> Switch1/1

== system part_m/scenario II/Lead Anggle1/Subsystem4/Subsystem2 ==
  epsilon : Inport
  sigma : Inport  Port=2
  delta_state : Inport  Port=3
  MATLAB Function : MATLAB Function  TreatAsAtomicUnit=on
  Product : Product  Multiplication=Matrix(*)
  Sqrt : Sqrt
  Transfer Fcn : TransferFcn  Numerator=[100 0]  Denominator=[1 100]
  Transfer Fcn2 : TransferFcn  Numerator=[100 0]  Denominator=[1 100]
  Transfer Fcn4 : TransferFcn  Numerator=[100 0]  Denominator=[1 100]
  Transpose : Math  Operator=transpose
  sigma phi : Outport
  epsilon phi : Outport  Port=2
  wires:
  sigma/1 -> Transfer Fcn/1
  Transfer Fcn/1 -> MATLAB Function/1(d_sigma)  "d_sigma"
  epsilon/1 -> Transfer Fcn2/1
  Transfer Fcn2/1 -> MATLAB Function/4(d_epsilon)  "d_epsilon"
  delta_state/1 -> Product/2, Transpose/1
  Product/1 -> Sqrt/1
  Transpose/1 -> Product/1
  Sqrt/1 -> MATLAB Function/3(delta_R), Transfer Fcn4/1  "R_m"
  Transfer Fcn4/1 -> MATLAB Function/2(d_delta_R)  "d_R_m"
  MATLAB Function/1(epsilon_phi) -> epsilon phi/1
  MATLAB Function/2(sigma_phi) -> sigma phi/1

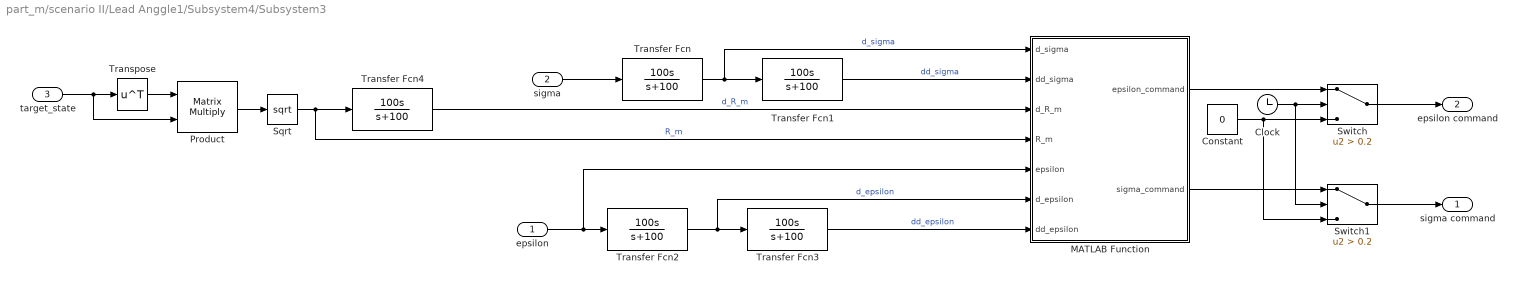
== system part_m/scenario II/Lead Anggle1/Subsystem4/Subsystem3 ==
  epsilon : Inport
  sigma : Inport  Port=2
  target_state : Inport  Port=3
  Clock : Clock
  Constant : Constant  Value=0
  MATLAB Function : MATLAB Function  TreatAsAtomicUnit=on
  Product : Product  Multiplication=Matrix(*)
  Sqrt : Sqrt
  Switch : Switch  Criteria=u2 > Threshold  Threshold=0.2  SaturateOnIntegerOverflow=off  InputSameDT=off
  Switch1 : Switch  Criteria=u2 > Threshold  Threshold=0.2  SaturateOnIntegerOverflow=off  InputSameDT=off
  Transfer Fcn{,1..4} (5 alike) : TransferFcn  Numerator=[100 0]  Denominator=[1 100]
  Transpose : Math  Operator=transpose
  sigma command : Outport
  epsilon command : Outport  Port=2
  wires:
  sigma/1 -> Transfer Fcn/1
  Transfer Fcn1/1 -> MATLAB Function/2(dd_sigma)  "dd_sigma"
  Transfer Fcn/1 -> MATLAB Function/1(d_sigma), Transfer Fcn1/1  "d_sigma"
  epsilon/1 -> MATLAB Function/5(epsilon), Transfer Fcn2/1
  Transfer Fcn2/1 -> MATLAB Function/6(d_epsilon), Transfer Fcn3/1  "d_epsilon"
  target_state/1 -> Product/2, Transpose/1
  Product/1 -> Sqrt/1
  Transpose/1 -> Product/1
  Sqrt/1 -> MATLAB Function/4(R_m), Transfer Fcn4/1  "R_m"
  Transfer Fcn3/1 -> MATLAB Function/7(dd_epsilon)  "dd_epsilon"
  Transfer Fcn4/1 -> MATLAB Function/3(d_R_m)  "d_R_m"
  Clock/1 -> Switch1/2, Switch/2
  Switch/1 -> epsilon command/1
  MATLAB Function/1(epsilon_command) -> Switch/1
  Constant/1 -> Switch1/3, Switch/3
  Switch1/1 -> sigma command/1
  MATLAB Function/2(sigma_command) -> Switch1/1

== system part_m/scenario III/Lead Anggle2/Subsystem4/Subsystem2 ==
  epsilon : Inport
  sigma : Inport  Port=2
  delta_state : Inport  Port=3
  MATLAB Function : MATLAB Function  TreatAsAtomicUnit=on
  Product : Product  Multiplication=Matrix(*)
  Sqrt : Sqrt
  Transfer Fcn : TransferFcn  Numerator=[100 0]  Denominator=[1 100]
  Transfer Fcn2 : TransferFcn  Numerator=[100 0]  Denominator=[1 100]
  Transfer Fcn4 : TransferFcn  Numerator=[100 0]  Denominator=[1 100]
  Transpose : Math  Operator=transpose
  sigma phi : Outport
  epsilon phi : Outport  Port=2
  wires:
  sigma/1 -> Transfer Fcn/1
  Transfer Fcn/1 -> MATLAB Function/1(d_sigma)  "d_sigma"
  epsilon/1 -> Transfer Fcn2/1
  Transfer Fcn2/1 -> MATLAB Function/4(d_epsilon)  "d_epsilon"
  delta_state/1 -> Product/2, Transpose/1
  Product/1 -> Sqrt/1
  Transpose/1 -> Product/1
  Sqrt/1 -> MATLAB Function/3(delta_R), Transfer Fcn4/1  "R_m"
  Transfer Fcn4/1 -> MATLAB Function/2(d_delta_R)  "d_R_m"
  MATLAB Function/1(epsilon_phi) -> epsilon phi/1
  MATLAB Function/2(sigma_phi) -> sigma phi/1

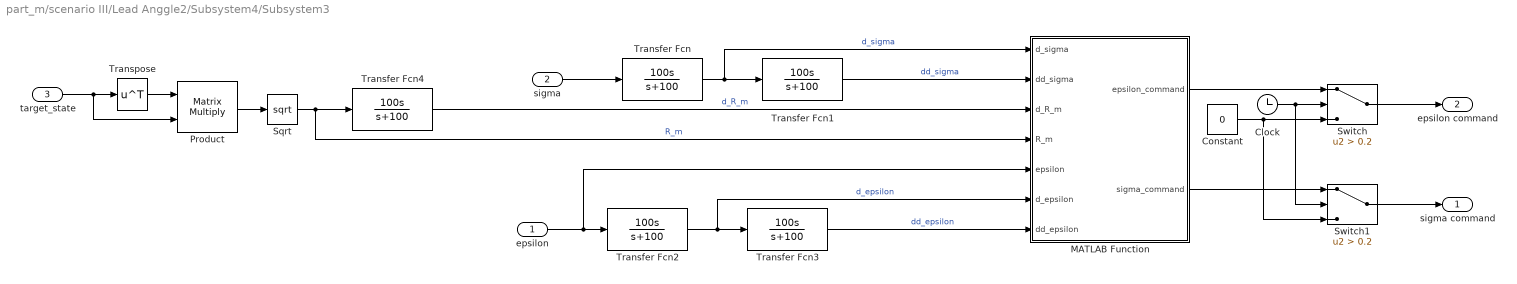
== system part_m/scenario III/Lead Anggle2/Subsystem4/Subsystem3 ==
  epsilon : Inport
  sigma : Inport  Port=2
  target_state : Inport  Port=3
  Clock : Clock
  Constant : Constant  Value=0
  MATLAB Function : MATLAB Function  TreatAsAtomicUnit=on
  Product : Product  Multiplication=Matrix(*)
  Sqrt : Sqrt
  Switch : Switch  Criteria=u2 > Threshold  Threshold=0.2  SaturateOnIntegerOverflow=off  InputSameDT=off
  Switch1 : Switch  Criteria=u2 > Threshold  Threshold=0.2  SaturateOnIntegerOverflow=off  InputSameDT=off
  Transfer Fcn{,1..4} (5 alike) : TransferFcn  Numerator=[100 0]  Denominator=[1 100]
  Transpose : Math  Operator=transpose
  sigma command : Outport
  epsilon command : Outport  Port=2
  wires:
  sigma/1 -> Transfer Fcn/1
  Transfer Fcn1/1 -> MATLAB Function/2(dd_sigma)  "dd_sigma"
  Transfer Fcn/1 -> MATLAB Function/1(d_sigma), Transfer Fcn1/1  "d_sigma"
  epsilon/1 -> MATLAB Function/5(epsilon), Transfer Fcn2/1
  Transfer Fcn2/1 -> MATLAB Function/6(d_epsilon), Transfer Fcn3/1  "d_epsilon"
  target_state/1 -> Product/2, Transpose/1
  Product/1 -> Sqrt/1
  Transpose/1 -> Product/1
  Sqrt/1 -> MATLAB Function/4(R_m), Transfer Fcn4/1  "R_m"
  Transfer Fcn3/1 -> MATLAB Function/7(dd_epsilon)  "dd_epsilon"
  Transfer Fcn4/1 -> MATLAB Function/3(d_R_m)  "d_R_m"
  Clock/1 -> Switch1/2, Switch/2
  Switch/1 -> epsilon command/1
  MATLAB Function/1(epsilon_command) -> Switch/1
  Constant/1 -> Switch1/3, Switch/3
  Switch1/1 -> sigma command/1
  MATLAB Function/2(sigma_command) -> Switch1/1

== matlab function part_m/scenario I/Target1/Transformation Matrix ==
  data: attitude input; T_GV output
function T_GV = fcn(attitude)
theta = attitude(1);
psi = attitude(2);

T_GV = [cos(theta)*cos(psi)   cos(theta)*sin(psi)   sin(theta)
            -sin(psi)               cos(psi)            0
        -sin(theta)*cos(psi)  -sin(theta)*sin(psi)   cos(theta) ];

== matlab function part_m/scenario I/Lead Anggle/Subsystem4/Subsystem3/MATLAB Function ==
  data: d_sigma input; dd_sigma input; d_R_m input; R_m input; epsilon input; d_epsilon input; dd_epsilon input; epsilon_command output; sigma_command output
function [epsilon_command, sigma_command] = fcn(d_sigma,dd_sigma, d_R_m, R_m, epsilon, d_epsilon, dd_epsilon)


epsilon_command = R_m*dd_epsilon + 2*d_R_m*d_epsilon ...
    + R_m*(d_sigma^2)*sin(epsilon)*cos(epsilon);


sigma_command   = (R_m*dd_sigma + 2*d_R_m*d_sigma)*cos(epsilon) ...
    - 2*R_m*d_epsilon*d_sigma*sin(epsilon);

== matlab function part_m/scenario II/Target2/MATLAB Function ==
  data: a input; dd_state output; V input; g_effect input; attitude input; dot_attitude output
function [dd_state, dot_attitude] =...
    fcn(a, V, g_effect, attitude)
a_x = a(1);
a_y = a(2);
a_z = a(3);

theta = attitude(1);
psi = attitude(2);
g = 9.81;
g = g*g_effect;

ddot_x = a_x*cos(theta)*cos(psi) - a_y*sin(psi) - a_z*sin(theta)*cos(psi);
ddot_y = a_x*cos(theta)*sin(psi) + a_y*cos(psi) - a_z*sin(theta)*sin(psi);
ddot_z = a_x*sin(theta) + a_z*cos(theta) - g;


dd_state = [ddot_x; ddot_y; ddot_z];

g = 9.81;
dot_theta = (a_z - g*cos(theta)) / V;
dot_psi   = a_y / (V*cos(theta));

dot_attitude = [dot_theta; dot_psi];

== matlab function part_m/scenario II/Target2/Transformation Matrix ==
  data: attitude input; T_GV output
function T_GV = fcn(attitude)
theta = attitude(1);
psi = attitude(2);

T_GV = [cos(theta)*cos(psi)   cos(theta)*sin(psi)   sin(theta)
            -sin(psi)               cos(psi)            0
        -sin(theta)*cos(psi)  -sin(theta)*sin(psi)   cos(theta) ];

== matlab function part_m/scenario I/Lead Anggle/MATLAB Function ==
  data: d_sigma output; missle_state input; d_epsilon output; target_state input; epsilon_t output; sigma_t output; sigma_phi input; epsilon_phi input
function [d_sigma, d_epsilon, epsilon_t, sigma_t] =...
    fcn(missle_state, target_state, sigma_phi, epsilon_phi)

[sigma_m, epsilon_m] = angle_calculator(missle_state);
[sigma_t, epsilon_t] = angle_calculator(target_state);

d_epsilon = norm(missle_state)*(epsilon_t - epsilon_m + epsilon_phi);
d_sigma = norm(missle_state)*(sigma_t - sigma_m + sigma_phi)*cos(epsilon_t+epsilon_phi);

end


function [sigma, epsilon] = angle_calculator(state)
    if norm(state) == 0
        epsilon = 0;
        sigma = 0;
        return
    end
    epsilon = asin(state(3)/norm(state));
    sigma = atan2(state(2),state(1));
end

== matlab function part_m/scenario I/Lead Anggle/MATLAB Function1 ==
  data: g_command output; target_state input
function g_command  = fcn(target_state)

[~, epsilon_t] = angle_calculator(target_state);
g = 9.81;
g_command = g * cos(epsilon_t);


end


function [sigma, epsilon] = angle_calculator(state)
    if norm(state) == 0
        epsilon = 0;
        sigma = 0;
        return
    end
    epsilon = asin(state(3)/norm(state));
    sigma = atan2(state(2),state(1));
end

== matlab function part_m/scenario I/Lead Anggle/Subsystem4/Subsystem2/MATLAB Function ==
  data: d_sigma input; d_delta_R input; delta_R input; d_epsilon input; epsilon_phi output; sigma_phi output
function [epsilon_phi, sigma_phi] = fcn(d_sigma, d_delta_R, delta_R, d_epsilon)


t_go = - delta_R / d_delta_R;
epsilon_phi = t_go * d_epsilon;


sigma_phi = t_go * d_sigma;

== matlab function part_m/scenario II/Lead Anggle1/MATLAB Function ==
  data: d_sigma output; missle_state input; d_epsilon output; target_state input; epsilon_t output; sigma_t output; sigma_phi input; epsilon_phi input
function [d_sigma, d_epsilon, epsilon_t, sigma_t] =...
    fcn(missle_state, target_state, sigma_phi, epsilon_phi)

[sigma_m, epsilon_m] = angle_calculator(missle_state);
[sigma_t, epsilon_t] = angle_calculator(target_state);

d_epsilon = norm(missle_state)*(epsilon_t - epsilon_m + epsilon_phi);
d_sigma = norm(missle_state)*(sigma_t - sigma_m + sigma_phi)*cos(epsilon_t+epsilon_phi);

end


function [sigma, epsilon] = angle_calculator(state)
    if norm(state) == 0
        epsilon = 0;
        sigma = 0;
        return
    end
    epsilon = asin(state(3)/norm(state));
    sigma = atan2(state(2),state(1));
end

== matlab function part_m/scenario III/Lead Anggle2/MATLAB Function ==
  data: d_sigma output; missle_state input; d_epsilon output; target_state input; epsilon_t output; sigma_t output; sigma_phi input; epsilon_phi input
function [d_sigma, d_epsilon, epsilon_t, sigma_t] =...
    fcn(missle_state, target_state, sigma_phi, epsilon_phi)

[sigma_m, epsilon_m] = angle_calculator(missle_state);
[sigma_t, epsilon_t] = angle_calculator(target_state);

d_epsilon = norm(missle_state)*(epsilon_t - epsilon_m + epsilon_phi);
d_sigma = norm(missle_state)*(sigma_t - sigma_m + sigma_phi)*cos(epsilon_t+epsilon_phi);

end


function [sigma, epsilon] = angle_calculator(state)
    if norm(state) == 0
        epsilon = 0;
        sigma = 0;
        return
    end
    epsilon = asin(state(3)/norm(state));
    sigma = atan2(state(2),state(1));
end

== matlab function part_m/scenario III/Lead Anggle2/MATLAB Function1 ==
  data: g_command output; target_state input
function g_command  = fcn(target_state)

[~, epsilon_t] = angle_calculator(target_state);
g = 9.81;
g_command = g * cos(epsilon_t);


end


function [sigma, epsilon] = angle_calculator(state)
    if norm(state) == 0
        epsilon = 0;
        sigma = 0;
        return
    end
    epsilon = asin(state(3)/norm(state));
    sigma = atan2(state(2),state(1));
end

== matlab function part_m/scenario III/Lead Anggle2/Subsystem4/Subsystem2/MATLAB Function ==
  data: d_sigma input; d_delta_R input; delta_R input; d_epsilon input; epsilon_phi output; sigma_phi output
function [epsilon_phi, sigma_phi] = fcn(d_sigma, d_delta_R, delta_R, d_epsilon)


t_go = - delta_R / d_delta_R;
epsilon_phi = t_go * d_epsilon;


sigma_phi = t_go * d_sigma;

== matlab function part_m/scenario III/Lead Anggle2/Subsystem4/Subsystem3/MATLAB Function ==
  data: d_sigma input; dd_sigma input; d_R_m input; R_m input; epsilon input; d_epsilon input; dd_epsilon input; epsilon_command output; sigma_command output
function [epsilon_command, sigma_command] = fcn(d_sigma,dd_sigma, d_R_m, R_m, epsilon, d_epsilon, dd_epsilon)


epsilon_command = R_m*dd_epsilon + 2*d_R_m*d_epsilon ...
    + R_m*(d_sigma^2)*sin(epsilon)*cos(epsilon);


sigma_command   = (R_m*dd_sigma + 2*d_R_m*d_sigma)*cos(epsilon) ...
    - 2*R_m*d_epsilon*d_sigma*sin(epsilon);

== matlab function part_m/scenario III/Missile 3/MATLAB Function ==
  data: a input; dd_state output; V input; g_effect input; attitude input; dot_attitude output
function [dd_state, dot_attitude] =...
    fcn(a, V, g_effect, attitude)
a_x = a(1);
a_y = a(2);
a_z = a(3);

theta = attitude(1);
psi = attitude(2);
g = 9.81;
g = g*g_effect;

ddot_x = a_x*cos(theta)*cos(psi) - a_y*sin(psi) - a_z*sin(theta)*cos(psi);
ddot_y = a_x*cos(theta)*sin(psi) + a_y*cos(psi) - a_z*sin(theta)*sin(psi);
ddot_z = a_x*sin(theta) + a_z*cos(theta) - g;

dd_state = [ddot_x; ddot_y; ddot_z];

dot_theta = (a_z - g*cos(theta)) / V;
dot_psi   = a_y / (V*cos(theta));

dot_attitude = [dot_theta; dot_psi];

== matlab function part_m/scenario III/Missile 3/Transformation Matrix ==
  data: attitude input; T_GV output
function T_GV = fcn(attitude)
theta = attitude(1);
psi = attitude(2);

T_GV = [cos(theta)*cos(psi)   cos(theta)*sin(psi)   sin(theta)
            -sin(psi)               cos(psi)            0
        -sin(theta)*cos(psi)  -sin(theta)*sin(psi)   cos(theta) ];

== matlab function part_m/scenario III/Target3/MATLAB Function ==
  data: a input; dd_state output; V input; g_effect input; attitude input; dot_attitude output
function [dd_state, dot_attitude] =...
    fcn(a, V, g_effect, attitude)
a_x = a(1);
a_y = a(2);
a_z = a(3);

theta = attitude(1);
psi = attitude(2);
g = 9.81;
g = g*g_effect;

ddot_x = a_x*cos(theta)*cos(psi) - a_y*sin(psi) - a_z*sin(theta)*cos(psi);
ddot_y = a_x*cos(theta)*sin(psi) + a_y*cos(psi) - a_z*sin(theta)*sin(psi);
ddot_z = a_x*sin(theta) + a_z*cos(theta) - g;


dd_state = [ddot_x; ddot_y; ddot_z];

g = 9.81;
dot_theta = (a_z - g*cos(theta)) / V;
dot_psi   = a_y / (V*cos(theta));

dot_attitude = [dot_theta; dot_psi];

== matlab function part_m/scenario III/Target3/Transformation Matrix ==
  data: attitude input; T_GV output
function T_GV = fcn(attitude)
theta = attitude(1);
psi = attitude(2);

T_GV = [cos(theta)*cos(psi)   cos(theta)*sin(psi)   sin(theta)
            -sin(psi)               cos(psi)            0
        -sin(theta)*cos(psi)  -sin(theta)*sin(psi)   cos(theta) ];
